simulink model "lab4_parall_sbl_2018b"  (R2018b)
settings: Solver=FixedStepAuto  StartTime=0.0  StopTime=100  FixedStep=0.05  RelTol=1e-3
libraries: simulink x2
settings Model: Creator=Olya Scherbak  LastModifiedBy=Танечка

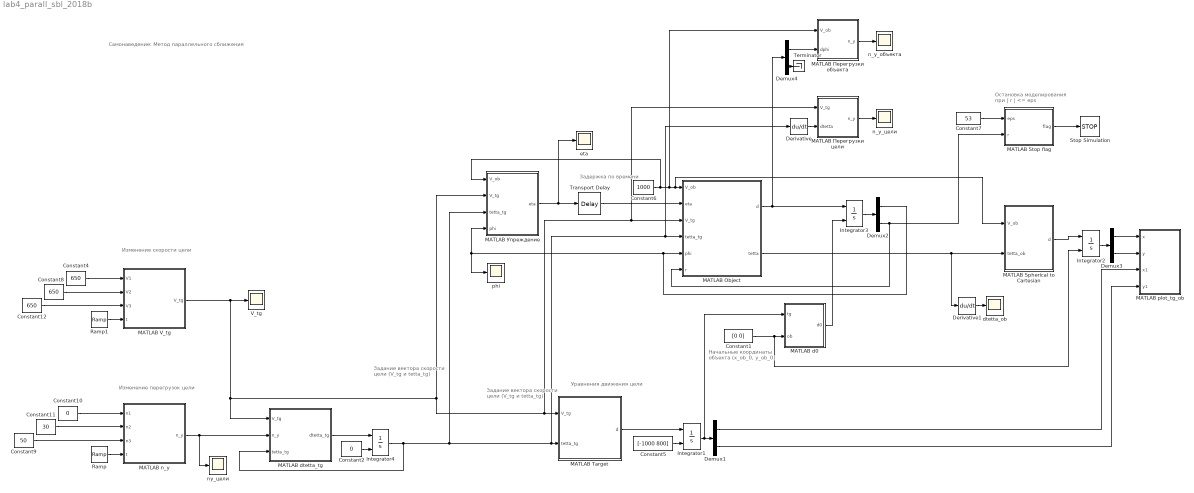
== system lab4_parall_sbl_2018b ==
  note: Задержка
      | по времени
  note: Изменение скорости цели
  note: Начальные координаты
      | объекта
      | (x_ob_0, y_ob_0)
  note: Остановка моделирования
      | при | r | <= eps
  note: Задание вектора
      | скорости цели
      | (V_tg и tetta_tg)
  note: Самонаведение: Метод параллельного сближения
  note: Уравнения
      | движения цели
  note: Задание вектора
      | скорости цели
      | (V_tg и tetta_tg)
  note: Изменение перегрузок цели
  Constant1 : Constant  Value=[0 0]  VectorParams1D=off
  Constant10 : Constant  Value=0
  Constant11 : Constant  Value=30
  Constant12 : Constant  Value=650
  Constant2 : Constant  Value=0
  Constant4 : Constant  Value=650
  Constant5 : Constant  Value=[-1000 800]  VectorParams1D=off
  Constant6 : Constant  Value=1000
  Constant7 : Constant  Value=53
  Constant8 : Constant  Value=650
  Constant9 : Constant  Value=50
  Demux{1..4} (4 alike) : Demux  Outputs=2
  Derivative : Derivative
  Derivative1 : Derivative
  Integrator{1..4} (4 alike) : Integrator  InitialConditionSource=external
  MATLAB Object : MATLAB Function  TreatAsAtomicUnit=on
  MATLAB Spherical to Cartesian : MATLAB Function  TreatAsAtomicUnit=on
  MATLAB Stop flag : MATLAB Function  TreatAsAtomicUnit=on
  MATLAB Target : MATLAB Function  TreatAsAtomicUnit=on
  MATLAB V_tg : MATLAB Function  TreatAsAtomicUnit=on
  MATLAB d0 : MATLAB Function  TreatAsAtomicUnit=on
  MATLAB dtetta_tg : MATLAB Function  TreatAsAtomicUnit=on
  MATLAB n_y : MATLAB Function  TreatAsAtomicUnit=on
  MATLAB plot_tg_ob : MATLAB Function  TreatAsAtomicUnit=on
  MATLAB Перегрузки объекта : MATLAB Function  TreatAsAtomicUnit=on
  MATLAB Перегрузки цели : MATLAB Function  TreatAsAtomicUnit=on
  MATLAB Упреждение : MATLAB Function  TreatAsAtomicUnit=on
  Ramp : simulink/Sources/Ramp  slope=2  start=0  InitialOutput=0
  Ramp1 : simulink/Sources/Ramp  slope=2  start=0  InitialOutput=0
  Stop Simulation : Stop
  Terminator : Terminator
  Transport Delay : TransportDelay  DelayTime=0.01
  V_tg : Scope
  dtetta_ob : Scope
  eta : Scope
  n_y_объекта : Scope
  n_y_цели : Scope
  ny_цели : Scope
  phi : Scope
  wires:
  MATLAB d0/1(d0) -> Integrator3/2
  Demux2/1 -> phi/1, MATLAB Упреждение/4(phi), MATLAB Object/5(phi)
  MATLAB Object/1(d) -> Demux4/1, Integrator3/1
  MATLAB Перегрузки цели/1(n_y) -> n_y_цели/1
  Demux1/1 -> MATLAB plot_tg_ob/3(x1)
  Integrator3/1 -> Demux2/1
  MATLAB Упреждение/1(eta) -> Transport Delay/1, eta/1
  Derivative/1 -> MATLAB Перегрузки цели/2(dtetta)
  Constant5/1 -> Integrator1/2
  MATLAB Target/1(d) -> Integrator1/1
  Constant7/1 -> MATLAB Stop flag/1(eps)
  Demux2/2 -> MATLAB Stop flag/2(r), MATLAB Object/6(r)
  MATLAB Stop flag/1(flag) -> Stop Simulation/1
  Constant6/1 -> MATLAB Spherical to Cartesian/1(V_ob), MATLAB Object/1(V_ob), MATLAB Перегрузки объекта/1(V_ob), MATLAB Упреждение/1(V_ob)
  Demux1/2 -> MATLAB plot_tg_ob/4(y1)
  MATLAB Object/2(tetta) -> Derivative1/1, MATLAB Spherical to Cartesian/2(tetta_ob)
  MATLAB Spherical to Cartesian/1(d) -> Integrator2/1
  Integrator1/1 -> MATLAB d0/1(tg), Demux1/1
  Integrator2/1 -> Demux3/1
  Demux3/1 -> MATLAB plot_tg_ob/1(x)
  Demux3/2 -> MATLAB plot_tg_ob/2(y)
  MATLAB n_y/1(n_y) -> MATLAB dtetta_tg/2(n_y), ny_цели/1
  Constant9/1 -> MATLAB n_y/3(n3)
  Constant11/1 -> MATLAB n_y/2(n2)
  Constant10/1 -> MATLAB n_y/1(n1)
  Ramp/1 -> MATLAB n_y/4(t)
  Constant1/1 -> MATLAB d0/2(ob), Integrator2/2
  MATLAB dtetta_tg/1(dtetta_tg) -> Integrator4/1
  Constant2/1 -> Integrator4/2
  Integrator4/1 -> MATLAB dtetta_tg/3(tetta_tg), MATLAB Упреждение/3(tetta_tg), Derivative/1, MATLAB Object/4(tetta_tg), MATLAB Target/2(tetta_tg)
  Demux4/1 -> MATLAB Перегрузки объекта/2(dphi)
  MATLAB Перегрузки объекта/1(n_y) -> n_y_объекта/1
  Constant4/1 -> MATLAB V_tg/1(V1)
  Constant12/1 -> MATLAB V_tg/3(V3)
  Ramp1/1 -> MATLAB V_tg/4(t)
  Constant8/1 -> MATLAB V_tg/2(V2)
  MATLAB V_tg/1(V_tg) -> MATLAB dtetta_tg/1(V_tg), MATLAB Перегрузки цели/1(V_tg), MATLAB Object/3(V_tg), MATLAB Target/1(V_tg), MATLAB Упреждение/2(V_tg), V_tg/1
  Demux4/2 -> Terminator/1
  Transport Delay/1 -> MATLAB Object/2(eta)
  Derivative1/1 -> dtetta_ob/1

== matlab function lab4_parall_sbl_2018b/MATLAB Target ==
  data: V_tg input; tetta_tg input; d output
function d   = Target(V_tg, tetta_tg)

% dx = V_tg*t*cos(tetta_tg); 
% dy = V_tg*t*sin(tetta_tg);

dx = V_tg*cos(tetta_tg); 
dy = V_tg*sin(tetta_tg);

d = [dx; dy];

end

== matlab function lab4_parall_sbl_2018b/MATLAB Упреждение ==
  data: V_ob input; V_tg input; tetta_tg input; phi input; eta output
function eta  = func(V_ob, V_tg, tetta_tg, phi)


        
 eta = asin((V_tg)*sin(phi - tetta_tg)/V_ob);
       
    
    

end

== matlab function lab4_parall_sbl_2018b/MATLAB d0 ==
  data: tg input; ob input; d0 output
function   d0 = func( tg, ob)

    x = tg(1) - ob(1);
    y = tg(2) - ob(2);

    phi_0 = atan2(y,x); 
    r_0   = sqrt(x^2 + y^2);

    d0 = [phi_0, r_0];

end

== matlab function lab4_parall_sbl_2018b/MATLAB dtetta_tg ==
  data: V_tg input; n_y input; tetta_tg input; dtetta_tg output
function dtetta_tg   = Target( V_tg, n_y, tetta_tg)

g = 9.81;

dtetta_tg = g*(n_y - cos(tetta_tg))/V_tg;

end

== matlab function lab4_parall_sbl_2018b/MATLAB Перегрузки цели ==
  data: V_tg input; dtetta input; n_y output
function n_y  = func( V_tg, dtetta)

g = 9.81;

n_y = V_tg*dtetta/g;


end

== matlab function lab4_parall_sbl_2018b/MATLAB Перегрузки объекта ==
  data: V_ob input; dphi input; n_y output
function n_y  = func( V_ob, dphi)

g = 9.81;

n_y = V_ob*dphi/g;


end

== matlab function lab4_parall_sbl_2018b/MATLAB n_y ==
  data: n1 input; n2 input; n3 input; n_y output; t input
function n_y   = Target(n1, n2, n3, t)

n_y = n1;

if (t>=0)&&(t<=0.7)
    n_y = n1;
end
if (t>0.7)&&(t<=1.5)
    n_y = n2;
end
if t>1.5
    n_y = n3;
end


end

== matlab function lab4_parall_sbl_2018b/MATLAB V_tg ==
  data: V1 input; V2 input; V3 input; V_tg output; t input
function V_tg  = Target(V1, V2, V3, t)

V_tg = V1;

if (t>=0)&&(t<=0.7)
    V_tg = V1;
end
if (t>0.7)&&(t<=1.5)
    V_tg = V2;
end
if t>1.5
    V_tg = V3;
end


end

== matlab function lab4_parall_sbl_2018b/MATLAB Object ==
  data: d output; V_ob input; eta input; V_tg input; tetta_tg input; phi input; r input; tetta output
function [d, tetta] = Object(V_ob, eta, V_tg, tetta_tg, phi, r)
    tetta = phi - eta;

    dr    =  -V_ob*cos(phi - tetta) + V_tg*cos(phi - tetta_tg);
    dphi  =  (V_ob*sin(phi - tetta))/r - (V_tg*sin(phi - tetta_tg))/r;
%     dphi  = 0;
   
    d = [dphi; dr];
end

== matlab function lab4_parall_sbl_2018b/MATLAB Spherical to Cartesian ==
  data: V_ob input; tetta_ob input; d output
function d = func(V_ob, tetta_ob)

% Из сферической системе координат в декартову

    dx = V_ob*cos(tetta_ob);
    dy = V_ob*sin(tetta_ob);             

    d = [dx, dy];

end

== matlab function lab4_parall_sbl_2018b/MATLAB plot_tg_ob ==
  data: x input; y input; x1 input; y1 input
function plot2d(x,y, x1, y1)

figure(3);
plot([x x1],[y y1],'k-');
hold on;
plot(x,y,'ob');
hold on;
plot(x1,y1,'or');
hold on;

xlabel('X');
ylabel('Y');


grid on;
grid minor;
axis('equal');
end

== matlab function lab4_parall_sbl_2018b/MATLAB Stop flag ==
  data: eps input; r input; flag output
function flag  = Stop_flag(eps, r)

flag = 0;

if abs(r) < eps
          flag = 1;          
end
     
end
